simulink model "Autonomic"  (Simulink 6.4)
settings: Solver=ode45  StartTime=0.0  StopTime=10.0  RelTol=1e-3
values from neighbouring files (symbols this model uses):
  fcs_zero = 25    [Respiratory_IC.m]
  fp_inf = 6.3    [Respiratory_IC.m]
  fp_zero = 3.2    [Respiratory_IC.m]
  fs_inf = 2.10    (= 2.1)    [Respiratory_IC.m]
  fs_zero = 16.11    [Respiratory_IC.m]
  k_p = 7.06    [Respiratory_IC.m]
  k_s = 0.07    [Respiratory_IC.m]
undefined symbols (not defined in the file or in its folder): theta_para_n
libraries: simulink x1
settings Model: LastModifiedBy=cPhonix
settings OptimizationCC: BlockReduction=off  BooleanDataType=off
settings DebuggingCC: SolverPrmCheckMsg=none  StrictBusMsg=None
settings HardwareCC: TargetUnknown=on

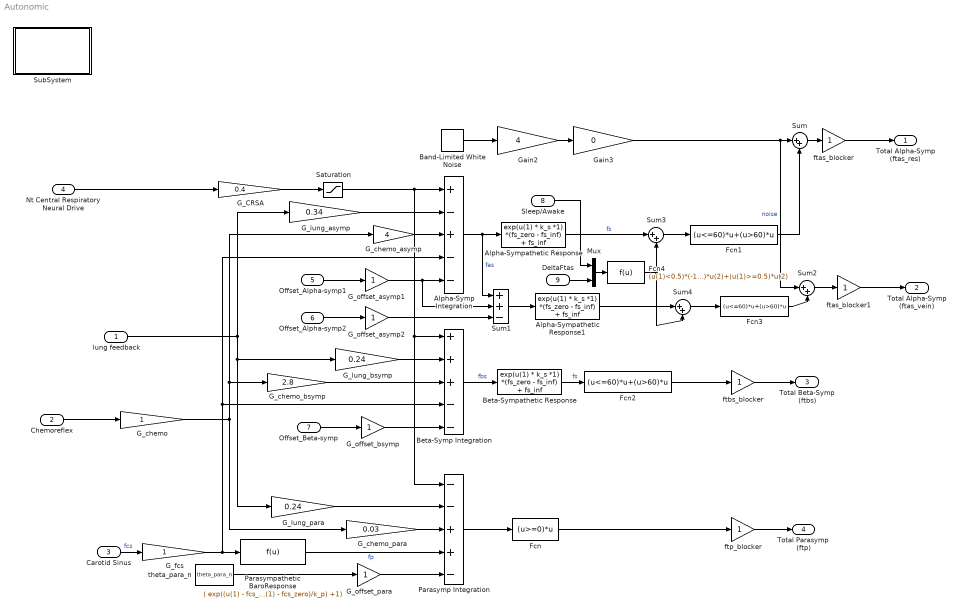
== system Autonomic ==
  lung feedback : Inport
  Chemoreflex : Inport  Port=2
  Carotid Sinus : Inport  Port=3
  Nt Central Respiratory Neural Drive : Inport  Port=4
  Offset_Alpha-symp1 : Inport  Port=5
  Offset_Alpha-symp2 : Inport  Port=6
  Offset_Beta-symp : Inport  Port=7
  Sleep/Awake : Inport  Port=8
  DeltaFtas : Inport  Port=9
  Alpha-Symp Integration : Sum  Inputs=+-+--  SaturateOnIntegerOverflow=on  InputSameDT=on
  Alpha-Sympathetic Response : Fcn  Expr=exp(u(1) * k_s *1) *(fs_zero - fs_inf) + fs_inf
  Alpha-Sympathetic Response1 : Fcn  Expr=exp(u(1) * k_s *1) *(fs_zero - fs_inf) + fs_inf
  Band-Limited White Noise : simulink/Sources/Band-Limited White Noise  SystemSampleTime=-1  Cov=[0.025]  Ts=0.1  seed=[23341]
  Beta-Symp Integration : Sum  Inputs=+++--  SaturateOnIntegerOverflow=on  InputSameDT=on
  Beta-Sympathetic Response : Fcn  Expr=exp(u(1) * k_s *1) *(fs_zero - fs_inf) + fs_inf
  Fcn : Fcn  Expr=(u>=0)*u
  Fcn1 : Fcn  Expr=(u<=60)*u+(u>60)*u
  Fcn2 : Fcn  Expr=(u<=60)*u+(u>60)*u
  Fcn3 : Fcn  Expr=(u<=60)*u+(u>60)*u
  Fcn4 : Fcn  Expr=(u(1)<0.5)*(-1)*u(2)+(u(1)>=0.5)*u(2)
  G_CRSA : Gain  Gain=0.4  SaturateOnIntegerOverflow=on
  G_chemo : Gain  SaturateOnIntegerOverflow=on
  G_chemo_asymp : Gain  Gain=4  SaturateOnIntegerOverflow=on
  G_chemo_bsymp : Gain  Gain=2.8  SaturateOnIntegerOverflow=on
  G_chemo_para : Gain  Gain=0.03  SaturateOnIntegerOverflow=on
  G_fcs : Gain  SaturateOnIntegerOverflow=on
  G_lung_asymp : Gain  Gain=0.34  SaturateOnIntegerOverflow=on
  G_lung_bsymp : Gain  Gain=0.24  SaturateOnIntegerOverflow=on
  G_lung_para : Gain  Gain=0.24  SaturateOnIntegerOverflow=on
  G_offset_asymp1 : Gain
  G_offset_asymp2 : Gain
  G_offset_bsymp : Gain
  G_offset_para : Gain
  Gain2 : Gain  Gain=4  SaturateOnIntegerOverflow=on
  Gain3 : Gain  Gain=0  SaturateOnIntegerOverflow=on
  Mux : Mux  Inputs=2
  "Parasymp Integration " : Sum  Inputs=--++-  SaturateOnIntegerOverflow=on  InputSameDT=on
  Parasympathetic BaroResponse : Fcn  Expr=( exp((u(1) - fcs_zero)/k_p) * fp_inf *1 + fp_zero) / (exp((u(1) - fcs_zero)/k_p) +1)
  Saturation : Saturate  UpperLimit=10  LowerLimit=-10
  SubSystem : Subsystem
      settings: OpenFcn=pneuma_variables
      mask Display: disp('"double click here"\n to load \nAutonomic \ninitial values');
  Sum{,2..4} (4 alike) : Sum  Inputs=|++  SaturateOnIntegerOverflow=on
  Sum1 : Sum  Inputs=++-  SaturateOnIntegerOverflow=on
  ftas_blocker : Gain  SaturateOnIntegerOverflow=on
  ftas_blocker1 : Gain  SaturateOnIntegerOverflow=on
  ftbs_blocker : Gain  SaturateOnIntegerOverflow=on
  ftp_blocker : Gain  SaturateOnIntegerOverflow=on
  theta_para_n : Constant  Value=theta_para_n  OutDataType=sfix(16)  ConRadixGroup=Use specified scaling  OutScaling=2^0  SampleTime=inf  FramePeriod=inf
  Total Alpha-Symp (ftas_res) : Outport
  Total Alpha-Symp (ftas_vein) : Outport  Port=2
  Total Beta-Symp (ftbs) : Outport  Port=3
  Total Parasymp (ftp) : Outport  Port=4
  wires:
  G_CRSA/1 -> Saturation/1
  Carotid Sinus/1 -> G_fcs/1  "fcs"
  "Parasymp Integration "/1 -> Fcn/1
  Beta-Symp Integration/1 -> Beta-Sympathetic Response/1  "fbs"
  lung feedback/1 -> G_lung_para/1, G_lung_bsymp/1, G_lung_asymp/1
  Chemoreflex/1 -> G_chemo/1
  Alpha-Symp Integration/1 -> Alpha-Sympathetic Response/1, Sum1/1  "fas"
  Fcn/1 -> ftp_blocker/1
  Beta-Sympathetic Response/1 -> Fcn2/1  "fs"
  Nt Central Respiratory Neural Drive/1 -> G_CRSA/1
  Parasympathetic BaroResponse/1 -> "Parasymp Integration "/4  "fp"
  G_chemo_para/1 -> "Parasymp Integration "/3
  G_lung_para/1 -> "Parasymp Integration "/2
  G_chemo_bsymp/1 -> Beta-Symp Integration/3
  G_lung_bsymp/1 -> Beta-Symp Integration/2
  G_lung_asymp/1 -> Alpha-Symp Integration/2
  G_chemo_asymp/1 -> Alpha-Symp Integration/3
  Band-Limited White Noise/1 -> Gain2/1
  Gain2/1 -> Gain3/1
  Gain3/1 -> Sum/1, Sum2/1  "noise"
  Sum/1 -> ftas_blocker/1
  Fcn2/1 -> ftbs_blocker/1
  Fcn1/1 -> Sum/2
  ftas_blocker/1 -> Total Alpha-Symp (ftas_res)/1
  ftbs_blocker/1 -> Total Beta-Symp (ftbs)/1
  ftp_blocker/1 -> Total Parasymp (ftp)/1
  Saturation/1 -> Alpha-Symp Integration/1, "Parasymp Integration "/1, Beta-Symp Integration/1
  G_fcs/1 -> Alpha-Symp Integration/4, Beta-Symp Integration/4, Parasympathetic BaroResponse/1
  Offset_Alpha-symp1/1 -> G_offset_asymp1/1
  Offset_Beta-symp/1 -> G_offset_bsymp/1
  theta_para_n/1 -> G_offset_para/1
  Offset_Alpha-symp2/1 -> G_offset_asymp2/1
  Fcn3/1 -> Sum2/2
  Sum2/1 -> ftas_blocker1/1
  ftas_blocker1/1 -> Total Alpha-Symp (ftas_vein)/1
  Sum1/1 -> Alpha-Sympathetic Response1/1
  G_offset_asymp1/1 -> Sum1/2, Alpha-Symp Integration/5
  G_offset_asymp2/1 -> Sum1/3
  G_offset_bsymp/1 -> Beta-Symp Integration/5
  G_offset_para/1 -> "Parasymp Integration "/5
  G_chemo/1 -> G_chemo_para/1, G_chemo_asymp/1, G_chemo_bsymp/1
  Alpha-Sympathetic Response/1 -> Sum3/1  "fs"
  Sum3/1 -> Fcn1/1
  Alpha-Sympathetic Response1/1 -> Sum4/1
  Sum4/1 -> Fcn3/1
  Fcn4/1 -> Sum3/2, Sum4/2
  Sleep/Awake/1 -> Mux/1
  Mux/1 -> Fcn4/1
  DeltaFtas/1 -> Mux/2

== system Autonomic/SubSystem ==
